simulink model "modeloSala"  (R2016b)
settings: Solver=ode45  StartTime=0.0  StopTime=2868  RelTol=1e-3
values from neighbouring files (symbols this model uses):
  ac = 370.96 / fator    (= 6.18266666667)    [carregaDadosDoModelo.m]
  ae = 329.2  / fator    (= 5.48666666667)    [carregaDadosDoModelo.m]    (also in carregaDadosSimulacao.m = 5.4867)
  ar = 1489   / fator    (= 24.8166666667)    [carregaDadosDoModelo.m]
  av = 414.17 / fator    (= 6.90283333333)    [carregaDadosDoModelo.m]    (also in carregaDadosSimulacao.m = 6.9028)
  K = 0.36783    [carregaDados.m]    (also in carregaDadosDoModelo.m = 0.01332; carregaDadosSimulacao.m = 0.01)
  Kc = 1       * fator    (= 60)    [carregaDadosDoModelo.m]    (also in carregaDadosSimulacao.m = 2.5)
  Ke = 0.395   * fator    (= 23.7)    [carregaDadosDoModelo.m]    (also in carregaDadosSimulacao.m = 1.4)
  Kp = 0.12    [carregaDados.m]    (also in carregaDadosSimulacao.m)
  Kr = 0.016835* fator    (= 1.0101)    [carregaDadosDoModelo.m]
  Kv = 0.647   * fator    (= 38.82)    [carregaDadosDoModelo.m]    (also in carregaDadosSimulacao.m = 3.3)
undefined symbols (not defined in the file or in its folder): ap
settings Model: Creator=root  LastModifiedBy=maripimentel
settings DataIOCC: LimitDataPoints=on  SaveFormat=Array
settings OptimizationCC: BlockReduction=off  BooleanDataType=off  LifeSpan=inf
settings DebuggingCC: SaveWithParameterizedLinksMsg=none  UnderspecifiedInitializationDetection=Classic  MergeDetectMultiDrivingBlocksExec=none  SignalResolutionControl=TryResolveAllWithWarning  SFUnexpectedBacktrackingDiag=warning  SFNoUnconditionalDefaultTransitionDiag=warning  SFExecutionAtInitializationDiag=none
settings HardwareCC: ProdBitPerPointer=32  ProdBitPerSizeT=32  ProdBitPerPtrDiffT=32  ProdLargestAtomicFloat=None  ProdIntDivRoundTo=Undefined  ProdEndianess=Unspecified  ProdWordSize=32  ProdHWDeviceType=32-bit Generic  TargetUnknown=on
settings ModelReferenceCC: PropagateSignalLabelsOutOfModel=off
settings GRTTargetCC: TargetLangStandard=C89/C90 (ANSI)  GeneratePreprocessorConditionals=Disable all
settings ConfigComp: CovMetricSettings=dw  CovHtmlReporting=on  CovSaveCumulativeToWorkspaceVar=on  CovSaveSingleToWorkspaceVar=on  CovExternalEMLEnable=off

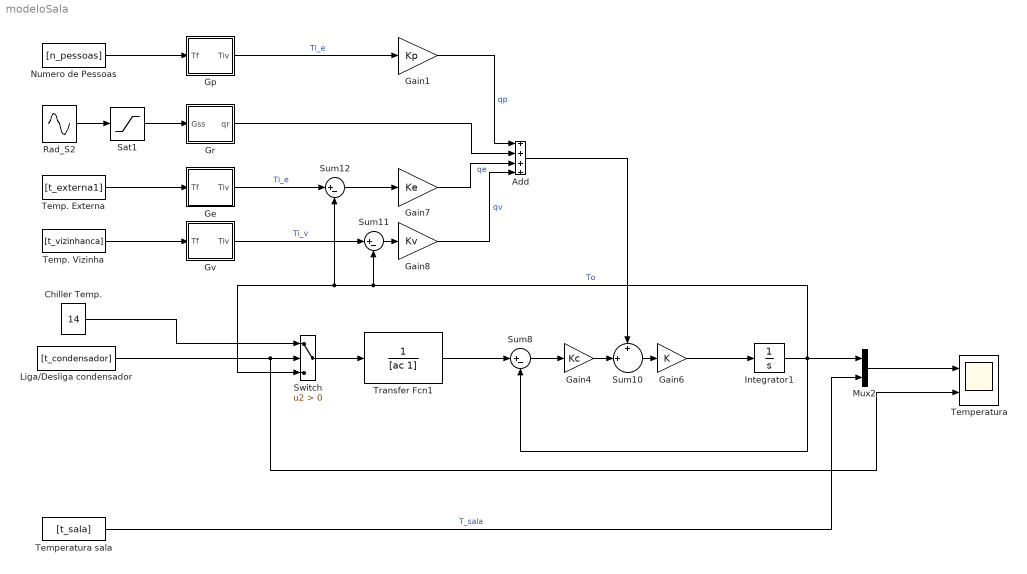
== system modeloSala ==
  Add : Sum  Inputs=++++
  Chiller Temp. : Constant  Value=14
  Gain1 : Gain  Gain=Kp
  Gain4 : Gain  Gain=Kc
  Gain6 : Gain  Gain=K
  Gain7 : Gain  Gain=Ke
  Gain8 : Gain  Gain=Kv
  Ge : Subsystem
  Gp : Subsystem
  Gr : Subsystem
  Gv : Subsystem
  Integrator1 : Integrator  InitialCondition=24
  Liga/Desliga condensador : FromWorkspace  VariableName=[t_condensador]  SampleTime=1
  Mux2 : Mux  Inputs=2
  Numero de Pessoas : FromWorkspace  VariableName=[n_pessoas]  SampleTime=1
  Rad_S2 : Sin  Amplitude=700  Frequency=2*pi/(24*60)  Phase=-pi/2-pi/3+pi  SampleTime=0
  Sat1 : Saturate  UpperLimit=1500  LowerLimit=0
  Sum10 : Sum  Inputs=+|+||
  Sum11 : Sum  Inputs=|+-
  Sum12 : Sum  Inputs=|+-
  Sum8 : Sum  Inputs=|+-
  Switch : Switch  Criteria=u2 > Threshold
  "Temp. Externa " : FromWorkspace  VariableName=[t_externa1]  SampleTime=1
  Temp. Vizinha : FromWorkspace  VariableName=[t_vizinhanca]  SampleTime=1
  Temperatura : Scope  NumInputPorts=2
  Temperatura sala : FromWorkspace  VariableName=[t_sala]  SampleTime=1
  Transfer Fcn1 : TransferFcn  Denominator=[ac 1]
  wires:
  Gain6/1 -> Integrator1/1
  Sum8/1 -> Gain4/1
  Gain4/1 -> Sum10/2
  Sum10/1 -> Gain6/1
  Sum12/1 -> Gain7/1
  Ge/1(Tiv) -> Sum12/1  "Ti_e"
  Integrator1/1 -> Switch/3, Sum12/2, Sum11/2, Mux2/1, Sum8/2  "To"
  Sum11/1 -> Gain8/1
  Gv/1(Tiv) -> Sum11/1  "Ti_v"
  Gain7/1 -> Add/3  "qe"
  Sat1/1 -> Gr/1(Gss)
  Gain8/1 -> Add/4  "qv"
  Rad_S2/1 -> Sat1/1
  Temp. Vizinha/1 -> Gv/1(Tf)
  Temperatura sala/1 -> Mux2/2  "T_sala"
  Add/1 -> Sum10/1
  Chiller Temp./1 -> Switch/1
  Liga/Desliga condensador/1 -> Switch/2, Temperatura/2
  Transfer Fcn1/1 -> Sum8/1
  "Temp. Externa "/1 -> Ge/1(Tf)
  Switch/1 -> Transfer Fcn1/1
  Mux2/1 -> Temperatura/1
  Gp/1(Tiv) -> Gain1/1  "Ti_e"
  Gr/1(qr) -> Add/2
  Numero de Pessoas/1 -> Gp/1(Tf)
  Gain1/1 -> Add/1  "qp"

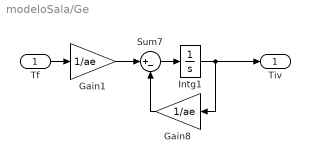
== system modeloSala/Ge ==
  Tf : Inport
  Gain1 : Gain  Gain=1/ae
  Gain8 : Gain  Gain=1/ae
  Intg1 : Integrator  InitialCondition=30
  Sum7 : Sum  Inputs=|+-
  Tiv : Outport
  wires:
  Gain1/1 -> Sum7/1
  Tf/1 -> Gain1/1
  Gain8/1 -> Sum7/2
  Intg1/1 -> Tiv/1, Gain8/1
  Sum7/1 -> Intg1/1

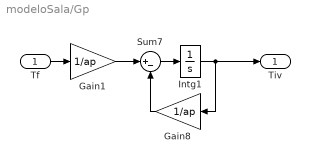
== system modeloSala/Gp ==
  Tf : Inport
  Gain1 : Gain  Gain=1/ap
  Gain8 : Gain  Gain=1/ap
  Intg1 : Integrator  InitialCondition=30
  Sum7 : Sum  Inputs=|+-
  Tiv : Outport
  wires:
  Gain1/1 -> Sum7/1
  Tf/1 -> Gain1/1
  Gain8/1 -> Sum7/2
  Intg1/1 -> Tiv/1, Gain8/1
  Sum7/1 -> Intg1/1

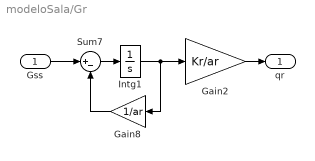
== system modeloSala/Gr ==
  Gss : Inport
  Gain2 : Gain  Gain=Kr/ar
  Gain8 : Gain  Gain=1/ar
  Intg1 : Integrator
  Sum7 : Sum  Inputs=|+-
  qr : Outport
  wires:
  Gain2/1 -> qr/1
  Gss/1 -> Sum7/1
  Gain8/1 -> Sum7/2
  Intg1/1 -> Gain2/1, Gain8/1
  Sum7/1 -> Intg1/1

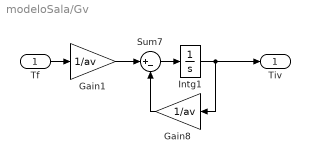
== system modeloSala/Gv ==
  Tf : Inport
  Gain1 : Gain  Gain=1/av
  Gain8 : Gain  Gain=1/av
  Intg1 : Integrator  InitialCondition=30
  Sum7 : Sum  Inputs=|+-
  Tiv : Outport
  wires:
  Gain1/1 -> Sum7/1
  Tf/1 -> Gain1/1
  Gain8/1 -> Sum7/2
  Intg1/1 -> Tiv/1, Gain8/1
  Sum7/1 -> Intg1/1
